simulink model "Grad4"  (R2016a)
settings: Solver=VariableStepAuto  StartTime=0.0  StopTime=1000000  RelTol=1e-3
values from neighbouring files (symbols this model uses):
  p = Primes(l)    [AlegePolinom.m]    (also in Top.m)
  Polinom = c(coeficient,:)    [AlegePolinom.m]    (also in Top.m = [c(1) c(2) c(3) c(4) c(5) c(6)])
  Seed = randi([1 p-1],[1 m])    [AlegePolinom.m]
settings Model: Creator=Orza  LastModifiedBy=Orza
settings DataIOCC: SaveTime=off

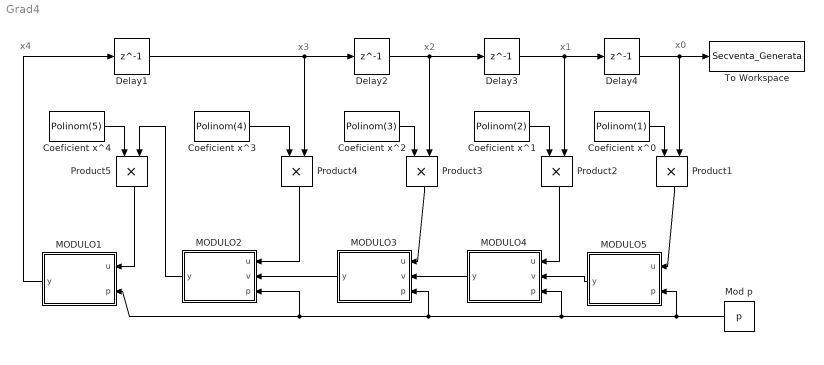
== system Grad4 ==
  note: x3
  note: x4
  note: x2
  note: x1
  note: x0
  Coeficient x^0 : Constant  Value=Polinom(1)
  Coeficient x^1 : Constant  Value=Polinom(2)
  Coeficient x^2 : Constant  Value=Polinom(3)
  Coeficient x^3 : Constant  Value=Polinom(4)
  Coeficient x^4 : Constant  Value=Polinom(5)
  Delay1 : Delay  DelayLength=1  InitialCondition=Seed(1)  SampleTime=1
  Delay2 : Delay  DelayLength=1  InitialCondition=Seed(2)  SampleTime=1
  Delay3 : Delay  DelayLength=1  InitialCondition=Seed(3)  SampleTime=1
  Delay4 : Delay  DelayLength=1  InitialCondition=Seed(4)  SampleTime=1
  MODULO1 : MATLAB Function  TreatAsAtomicUnit=on
  MODULO2 : MATLAB Function  TreatAsAtomicUnit=on
  MODULO3 : MATLAB Function  TreatAsAtomicUnit=on
  MODULO4 : MATLAB Function  TreatAsAtomicUnit=on
  MODULO5 : MATLAB Function  TreatAsAtomicUnit=on
  Mod p : Constant  Value=p
  Product{1..5} (5 alike) : Product
  To Workspace : ToWorkspace  VariableName=Secventa_Generata  SampleTime=-1
      settings: Save2DSignal=2-D array (concatenate along first dimension)
  wires:
  Delay4/1 -> Product1/2, To Workspace/1
  Delay3/1 -> Product2/2, Delay4/1
  Delay2/1 -> Delay3/1, Product3/2
  Product5/1 -> MODULO1/1(u)
  Coeficient x^4/1 -> Product5/1
  Product3/1 -> MODULO3/1(u)
  Coeficient x^2/1 -> Product3/1
  MODULO4/1(y) -> MODULO3/2(v)
  Product2/1 -> MODULO4/1(u)
  MODULO5/1(y) -> MODULO4/2(v)
  Product1/1 -> MODULO5/1(u)
  Mod p/1 -> MODULO5/2(p), MODULO4/3(p), MODULO3/3(p), MODULO2/3(p), MODULO1/2(p)
  Product4/1 -> MODULO2/1(u)
  MODULO3/1(y) -> MODULO2/2(v)
  Delay1/1 -> Product4/2, Delay2/1
  MODULO1/1(y) -> Delay1/1
  MODULO2/1(y) -> Product5/2
  Coeficient x^3/1 -> Product4/1
  Coeficient x^0/1 -> Product1/1
  Coeficient x^1/1 -> Product2/1

== matlab function Grad4/MODULO2 ==
  data: u input; y output; v input; p input
function y = fcn(u,v,p)
%#codegen

y = mod(u+v,p);

== matlab function Grad4/MODULO1 ==
  data: u input; y output; p input
function y = fcn(u,p)
%#codegen

y = mod(u,p);

== matlab function Grad4/MODULO3 ==
  data: u input; y output; v input; p input
function y = fcn(u,v,p)
%#codegen

y = mod(u+v,p);

== matlab function Grad4/MODULO4 ==
  data: u input; y output; v input; p input
function y = fcn(u,v,p)
%#codegen

y = mod(u+v,p);

== matlab function Grad4/MODULO5 ==
  data: u input; y output; p input
function y = fcn(u,p)
%#codegen

y = mod(u,p);
